simulink model "DemonstratorSimscape"  (R2020b)
settings: Solver=ode113  StartTime=0.0  StopTime=t_stop*0+20  FixedStep=1e-4
values from neighbouring files (symbols this model uses):
  brkD = 0    [main.m]
  brkI = 1e4    (= 10000)    [main.m]
  brkP = 1e5    (= 100000)    [main.m]
  d_drm = 0.5*d_drum    [main.m]
  d_shm = 0.4*d_sheave    [main.m]
  DeltaCable0 = 0    [main.m]
  Droop_scaling = 0    [main.m]
  eta_sh = 0.015    [main.m]
  filt_NUM = ones(1,200)*0.005    [main.m]
  g = 9.80665    [main.m]
  Iw = 0.5*(W.i + M.in*GB.r^2)    [main.m]
  Kp_mul = 0.3    [main.m]
  Lc0 = abs((T.ph-L.height-P.d-L.z0)*0.001)    [main.m]
  Ls1 = ((T.ph-0.5*W.pd)/1000)    [main.m]
  Ls2 = ((0.5*(T.s2+P.d)-2*P.d)/1000)    [main.m]
  M = 50e3    (= 50000)    [calcGrav.m]
  phi0_drm = -90    [main.m]
  phi0_shm = -90    [main.m]
  r_sheave = P.d*0.5    [main.m]
  s = tf('s')    [calcGrav.m]
  tau_brk = 0.001    [main.m]
  tau_em = 60e-3    (= 0.06)    [calcGrav.m]    (also in main.m)
  tau_m = tau_w/GB.r    [main.m]
  Tmax = 400e3    (= 400000)    [main.m]
  Tn_mul = 10    [main.m]
  x_drm = 0.7*r_drum    [main.m]
  x_shm = 0.7*r_sheave    [main.m]
  z0 = 0    [calcGrav.m]    (also in main.m = L.z0-P.d*0.5-P.d-P.d-L.height-T.h1-T.h2-32)
undefined symbols (not defined in the file or in its folder): C, CA, Controller_sampleTime, DiscIntNeverNeededParam, GB, L, P, Part, T, VFD_acceleration_model_factor, VFD_Adapt_factor_lower_p1458, VFD_Adapt_factor_upper_p1459, VFD_Curr_limit_var_p0641, VFD_Current_limit_p0640, VFD_Id_setp_total_r1624, VFD_Iq, VFD_Kp_n_basic_p1460, VFD_M, VFD_M_accel_T_smooth_p1517, VFD_M_lim_var_fixS_src_p1551, VFD_M_max_lower_p1521, VFD_M_max_lower_scal_p1525, VFD_M_max_up_mot_scal_p1524, VFD_M_max_upper_p1520, VFD_n_act_T_smooth_p1442, VFD_n_ctr_Kp_n_up_scal_p1461, VFD_n_ctr_Tn_n_up_sca_p1463, VFD_n_ctrl_adapt_Kp_lower_p1456, VFD_n_ctrl_adapt_Kp_upper_p1457, VFD_n_ctrl_Adpt_sig_Kp_p1455, VFD_n_ctrl_Kp_scal_p1466, VFD_n_ctrl_n_lower_p1464, VFD_n_ctrl_n_upper_p1465, VFD_n_ctrl_Tn_n_lower_p1462, VFD_n_limit_neg_p1086, VFD_n_limit_pos_p1083, VFD_n_limit_setp_p1063, VFD_n_max_p1082, VFD_n_set_filt_1_T_p1416, VFD_P_max_gen_p1531, VFD_P_max_mot_p1530, VFD_PU_I_outp_max_r0289, VFD_RFG_ramp_down_time_p1121, VFD_RFG_ramp_up_time_p1120, VFD_RFG_t_RD_scal_p1139, VFD_RFG_t_RU_scal_p1138, VSD, W, X, Y, Z
libraries: sm_lib x248, nesl_utility x128, simulink x49, pid_lib x4, cstblocks x2, simulink_extras x2
(part 5 of 10)

== system DemonstratorSimscape/Transmission System/Roof Pulley Set/Sheave_04 ==
  " " : sm_lib/Frames and Transforms/Rigid Transform  TranslationMethod=Cartesian  TranslationStandardOffset=0  TranslationLengthUnit=mm  TranslationStandardAxis=+Z  TranslationCartesianOffset=[0 -P.Bd*.25 -P.h]  TranslationROffset=0  TranslationROffsetUnits=m  TranslationZOffset=0  TranslationZOffsetUnits=m  TranslationThetaOffset=0  TranslationThetaOffsetUnits=deg  RotationMethod=ArbitraryAxis  RotationAngleUnits=deg  RotationStandardAxis=+Z  RotationAngle=90  RotationArbitraryAxis=[1 0 0]  FollAlignAxisA=+X  BaseAlignAxisA=+Y  FollAlignAxisB=+Y  BaseAlignAxisB=+Z  RotationSequenceAxes=FollowerAxes  RotationSequence=XYX  RotationSequenceAngles=[0 0 0]  RotationSequenceAnglesUnits=deg  RotationMatrix=[1 0 0; 0 1 0; 0 0 1]
  " 4" : sm_lib/Frames and Transforms/Rigid Transform  TranslationMethod=Cartesian  TranslationStandardOffset=0  TranslationLengthUnit=mm  TranslationStandardAxis=+Z  TranslationCartesianOffset=[0 -P.Bd*.25 P.h]  TranslationROffset=0  TranslationROffsetUnits=m  TranslationZOffset=0  TranslationZOffsetUnits=m  TranslationThetaOffset=0  TranslationThetaOffsetUnits=deg  RotationMethod=ArbitraryAxis  RotationAngleUnits=deg  RotationStandardAxis=+Z  RotationAngle=90  RotationArbitraryAxis=[1 0 0]  FollAlignAxisA=+X  BaseAlignAxisA=+Y  FollAlignAxisB=+Y  BaseAlignAxisB=+Z  RotationSequenceAxes=FollowerAxes  RotationSequence=XYX  RotationSequenceAngles=[0 0 0]  RotationSequenceAnglesUnits=deg  RotationMatrix=[1 0 0; 0 1 0; 0 0 1]
  PS>Sim1 : Subsystem
  Pulley 5 : sm_lib/Belts and Cables/Pulley  PitchRadius=P.Bd*0.5  PitchRadiusUnits=mm  InitialWrapAngleLowerBound=0.0  InitialWrapAngleLowerBoundUnits=deg  SenseWrapAngle=off  SensePulleyAngleA=off  SensePulleyAngleB=off  SenseFleetAngleA=off  SenseFleetAngleB=off
      settings: SourceProductBaseCode=MS
  Pulley rught red2 : Subsystem
      mask Display: image('sm_cable_drive_right_angle_pulleyA_IMAGE.png');
  Revolute Pulley5 : sm_lib/Joints/Revolute Joint  JointMode=Normal  SenseConstraintForce=on  SenseConstraintForceX=off  SenseConstraintForceY=off  SenseConstraintForceZ=off  SenseConstraintTorque=on  SenseConstraintTorqueX=off  SenseConstraintTorqueY=off  SenseConstraintTorqueZ=off  SenseTotalForce=on  SenseTotalForceX=off  SenseTotalForceY=off  SenseTotalForceZ=off  SenseTotalTorque=on  SenseTotalTorqueX=off  SenseTotalTorqueY=off  SenseTotalTorqueZ=off  CompositeWrenchDir=FollowerOnBase  CompositeWrenchFrame=BaseFrame  EquilibriumPosition=0  EquilibriumPositionUnits=deg  SpringStiffness=0  SpringStiffnessUnits=N*m/deg  DampingCoefficient=b_pulley  DampingCoefficientUnits=N*m/(deg/s)  TorqueActuationMode=NoTorque  MotionActuationMode=ComputedMotion  SensePosition=on  SenseVelocity=on  SenseAcceleration=on  SenseTorqueForce=on  SenseLowerLimitTorqueForce=off  SenseUpperLimitTorqueForce=off  LowerLimitSpecify=off  LowerLimitBound=-90  LowerLimitBoundUnits=deg  LowerLimitStiffness=1e4  LowerLimitStiffnessUnits=N*m/deg  LowerLimitDamping=10  LowerLimitDampingUnits=N*m/(deg/s)  LowerLimitTransitionRegionWidth=0.1  LowerLimitTransitionRegionWidthUnits=deg  UpperLimitSpecify=off  UpperLimitBound=90  UpperLimitBoundUnits=deg  UpperLimitStiffness=1e4  UpperLimitStiffnessUnits=N*m/deg  UpperLimitDamping=10  UpperLimitDampingUnits=N*m/(deg/s)  UpperLimitTransitionRegionWidth=0.1  UpperLimitTransitionRegionWidthUnits=deg  PositionTargetSpecify=off  PositionTargetPriority=High  PositionTargetValue=0  PositionTargetValueUnits=deg  VelocityTargetSpecify=off  VelocityTargetPriority=High  VelocityTargetValue=0  VelocityTargetValueUnits=deg/s
  ScopePulley5 : Scope  Commented=on  NumInputPorts=8
  Solid : sm_lib/Body Elements/Spherical Solid  GraphicAmbientColor=[0.15 0.15 0.15 1.0]  BasedOnType=Mass  CenterOfMass=[0 0 0]  CenterOfMassUnits=m  GraphicDiffuseColor=[0.5 0.5 0.5]  Density=1000  DensityUnits=kg/m^3  DoExposeReferenceFrame=on  GraphicEmissiveColor=[0.0 0.0 0.0 1.0]  ExportEntireGeometry=off  SerializedExposedGeometries=<ExposedGeometries/>  SerializedFrames=<Frames/>  MarkerShape=Sphere  MarkerSize=10  GraphicType=FromGeometry  InertiaType=CalculateFromGeometry  Mass=0.01  MassUnits=kg  MomentsOfInertia=[1 1 1]  MomentsOfInertiaUnits=kg*m^2  GraphicOpacity=1.0  ProductsOfInertia=[0 0 0]  ProductsOfInertiaUnits=kg*m^2  GraphicShininess=75  GraphicSpecularColor=[0.5 0.5 0.5 1.0]  SphereRadius=0.00001  SphereRadiusUnits=m  GraphicVisPropType=SimpleVisualProperties
  left face : sm_lib/Body Elements/Brick Solid  GraphicAmbientColor=[0.15 0.15 0.15 1.0]  BasedOnType=Density  BrickDimensions=[P.Bd P.h P.Bd*.5]  BrickDimensionUnits=mm  CenterOfMass=[0 0 0]  CenterOfMassUnits=m  GraphicDiffuseColor=[0.6 0.6 0.0]  Density=0  DensityUnits=g/cm^3  DoExposeReferenceFrame=on  GraphicEmissiveColor=[0.0 0.0 0.0 1.0]  ExportEntireGeometry=off  SerializedFrames=<Frames/>  MarkerShape=Sphere  MarkerSize=10  GraphicType=FromGeometry  InertiaType=CalculateFromGeometry  Mass=1  MassUnits=kg  MomentsOfInertia=[1 1 1]  MomentsOfInertiaUnits=kg*m^2  GraphicOpacity=c.opac  ProductsOfInertia=[0 0 0]  ProductsOfInertiaUnits=kg*m^2  GraphicShininess=75  GraphicSpecularColor=[0.5 0.5 0.5 1.0]  GraphicVisPropType=SimpleVisualProperties
  right face : sm_lib/Body Elements/Brick Solid  GraphicAmbientColor=[0.15 0.15 0.15 1.0]  BasedOnType=Density  BrickDimensions=[P.Bd P.h P.Bd*.5]  BrickDimensionUnits=mm  CenterOfMass=[0 0 0]  CenterOfMassUnits=m  GraphicDiffuseColor=[0.6 0.6 0.0]  Density=0  DensityUnits=g/cm^3  DoExposeReferenceFrame=on  GraphicEmissiveColor=[0.0 0.0 0.0 1.0]  ExportEntireGeometry=off  SerializedFrames=<Frames/>  MarkerShape=Sphere  MarkerSize=10  GraphicType=FromGeometry  InertiaType=CalculateFromGeometry  Mass=1  MassUnits=kg  MomentsOfInertia=[1 1 1]  MomentsOfInertiaUnits=kg*m^2  GraphicOpacity=1.0  ProductsOfInertia=[0 0 0]  ProductsOfInertiaUnits=kg*m^2  GraphicShininess=75  GraphicSpecularColor=[0.5 0.5 0.5 1.0]  GraphicVisPropType=SimpleVisualProperties
  w (rad/s) : nesl_utility/PS-Simulink Converter  PhysicalDomain=network_engine_domain  SubClassName=ps_output  LeftPortType=input  RightPortType=output  PseudoPeriodic=off  Frequencies=[]  Unit=rad/s  AffineConversion=off
  B : PMIOPort  Side=Left
  WireB : PMIOPort  Port=2  Side=Right
  WireA : PMIOPort  Port=3  Side=Right
  w5 : Outport  VectorParamsAs1DForOutWhenUnconnected=off
  wires:
  PS>Sim1/6(Out6) -> ScopePulley5/6
  PS>Sim1/3(Out3) -> ScopePulley5/3
  PS>Sim1/2(Out2) -> ScopePulley5/2
  PS>Sim1/1(Out1) -> ScopePulley5/1
  PS>Sim1/8(Out8) -> ScopePulley5/8
  PS>Sim1/7(Out7) -> ScopePulley5/7
  PS>Sim1/4(Out4) -> ScopePulley5/4
  PS>Sim1/5(Out5) -> ScopePulley5/5
  w (rad/s)/1 -> w5/1
  connections:
  " "/LConn1 -- B/RConn1 -- Revolute Pulley5/LConn1 -- " 4"/LConn1
  Solid/RConn1 -- Revolute Pulley5/RConn1 -- Pulley rught red2/LConn1
  Revolute Pulley5/RConn6 -- PS>Sim1/LConn5
  Revolute Pulley5/RConn4 -- PS>Sim1/LConn3
  Revolute Pulley5/RConn7 -- PS>Sim1/LConn6
  Revolute Pulley5/RConn5 -- PS>Sim1/LConn4
  Revolute Pulley5/RConn9 -- PS>Sim1/LConn8
  Revolute Pulley5/RConn8 -- PS>Sim1/LConn7
  Revolute Pulley5/RConn3 -- w (rad/s)/LConn1 -- PS>Sim1/LConn2
  Revolute Pulley5/RConn2 -- PS>Sim1/LConn1
  " 4"/RConn1 -- left face/RConn1
  " "/RConn1 -- right face/RConn1
  WireB/RConn1 -- Pulley 5/RConn2
  Pulley rught red2/RConn1 -- Pulley 5/LConn1
  WireA/RConn1 -- Pulley 5/RConn1

== system DemonstratorSimscape/Transmission System/Roof Pulley Set/Sheave_06 ==
  " " : sm_lib/Frames and Transforms/Rigid Transform  TranslationMethod=Cartesian  TranslationStandardOffset=0  TranslationLengthUnit=mm  TranslationStandardAxis=+Z  TranslationCartesianOffset=[0 -P.d*.25 -P.h]  TranslationROffset=0  TranslationROffsetUnits=m  TranslationZOffset=0  TranslationZOffsetUnits=m  TranslationThetaOffset=0  TranslationThetaOffsetUnits=deg  RotationMethod=ArbitraryAxis  RotationAngleUnits=deg  RotationStandardAxis=+Z  RotationAngle=90  RotationArbitraryAxis=[1 0 0]  FollAlignAxisA=+X  BaseAlignAxisA=+Y  FollAlignAxisB=+Y  BaseAlignAxisB=+Z  RotationSequenceAxes=FollowerAxes  RotationSequence=XYX  RotationSequenceAngles=[0 0 0]  RotationSequenceAnglesUnits=deg  RotationMatrix=[1 0 0; 0 1 0; 0 0 1]
  " 4" : sm_lib/Frames and Transforms/Rigid Transform  TranslationMethod=Cartesian  TranslationStandardOffset=0  TranslationLengthUnit=mm  TranslationStandardAxis=+Z  TranslationCartesianOffset=[0 -P.d*.25 P.h]  TranslationROffset=0  TranslationROffsetUnits=m  TranslationZOffset=0  TranslationZOffsetUnits=m  TranslationThetaOffset=0  TranslationThetaOffsetUnits=deg  RotationMethod=ArbitraryAxis  RotationAngleUnits=deg  RotationStandardAxis=+Z  RotationAngle=90  RotationArbitraryAxis=[1 0 0]  FollAlignAxisA=+X  BaseAlignAxisA=+Y  FollAlignAxisB=+Y  BaseAlignAxisB=+Z  RotationSequenceAxes=FollowerAxes  RotationSequence=XYX  RotationSequenceAngles=[0 0 0]  RotationSequenceAnglesUnits=deg  RotationMatrix=[1 0 0; 0 1 0; 0 0 1]
  Bending loss : Subsystem  Commented=on
  Constant : Constant  Value=g*1000
  Demux : Demux  Outputs=3
  Divide : Product  Inputs=*/
  Gain : Gain
  Gain1 : Gain  Gain=-2
  Nm : nesl_utility/Simulink-PS Converter  PhysicalDomain=network_engine_domain  SubClassName=ps_input  LeftPortType=input  RightPortType=output  PseudoPeriodic=off  Frequencies=[]  NoiseDistribution=none  NoiseParameters=[]  Unit=1  AffineConversion=off  FilteringAndDerivatives=filter  SimscapeFilterOrder=2  InputFilterTimeConstant=tau_bending  UdotUserProvided=0
  PS>Sim1 : Subsystem
  Pulley 6 : sm_lib/Belts and Cables/Pulley  PitchRadius=P.d*0.5  PitchRadiusUnits=mm  InitialWrapAngleLowerBound=0.0  InitialWrapAngleLowerBoundUnits=deg  SenseWrapAngle=off  SensePulleyAngleA=off  SensePulleyAngleB=off  SenseFleetAngleA=off  SenseFleetAngleB=off
      settings: SourceProductBaseCode=MS
  Revolute Pulley6 : sm_lib/Joints/Revolute Joint  JointMode=Normal  SenseConstraintForce=on  SenseConstraintForceX=off  SenseConstraintForceY=off  SenseConstraintForceZ=off  SenseConstraintTorque=on  SenseConstraintTorqueX=off  SenseConstraintTorqueY=off  SenseConstraintTorqueZ=off  SenseTotalForce=on  SenseTotalForceX=off  SenseTotalForceY=off  SenseTotalForceZ=off  SenseTotalTorque=on  SenseTotalTorqueX=off  SenseTotalTorqueY=off  SenseTotalTorqueZ=off  CompositeWrenchDir=FollowerOnBase  CompositeWrenchFrame=BaseFrame  EquilibriumPosition=0  EquilibriumPositionUnits=deg  SpringStiffness=0  SpringStiffnessUnits=N*m/deg  DampingCoefficient=b_pulley  DampingCoefficientUnits=N*m/(deg/s)  TorqueActuationMode=InputTorque  MotionActuationMode=ComputedMotion  SensePosition=on  SenseVelocity=on  SenseAcceleration=on  SenseTorqueForce=on  SenseLowerLimitTorqueForce=off  SenseUpperLimitTorqueForce=off  LowerLimitSpecify=off  LowerLimitBound=-90  LowerLimitBoundUnits=deg  LowerLimitStiffness=1e4  LowerLimitStiffnessUnits=N*m/deg  LowerLimitDamping=10  LowerLimitDampingUnits=N*m/(deg/s)  LowerLimitTransitionRegionWidth=0.1  LowerLimitTransitionRegionWidthUnits=deg  UpperLimitSpecify=off  UpperLimitBound=90  UpperLimitBoundUnits=deg  UpperLimitStiffness=1e4  UpperLimitStiffnessUnits=N*m/deg  UpperLimitDamping=10  UpperLimitDampingUnits=N*m/(deg/s)  UpperLimitTransitionRegionWidth=0.1  UpperLimitTransitionRegionWidthUnits=deg  PositionTargetSpecify=off  PositionTargetPriority=High  PositionTargetValue=0  PositionTargetValueUnits=deg  VelocityTargetSpecify=off  VelocityTargetPriority=High  VelocityTargetValue=0  VelocityTargetValueUnits=deg/s
  ScopePulley6 : Scope  Commented=on  NumInputPorts=8
  Sheave6 : Subsystem
      mask Display: image('sm_cable_drive_right_angle_pulleyA_IMAGE.png');
  left face : sm_lib/Body Elements/Brick Solid  GraphicAmbientColor=[0.15 0.15 0.15 1.0]  BasedOnType=Density  BrickDimensions=[P.d P.h P.d*.5]  BrickDimensionUnits=mm  CenterOfMass=[0 0 0]  CenterOfMassUnits=m  GraphicDiffuseColor=[0.6 0.6 0.0]  Density=0  DensityUnits=g/cm^3  DoExposeReferenceFrame=on  GraphicEmissiveColor=[0.0 0.0 0.0 1.0]  ExportEntireGeometry=off  SerializedFrames=<Frames/>  MarkerShape=Sphere  MarkerSize=10  GraphicType=FromGeometry  InertiaType=CalculateFromGeometry  Mass=1  MassUnits=kg  MomentsOfInertia=[1 1 1]  MomentsOfInertiaUnits=kg*m^2  GraphicOpacity=c.opac  ProductsOfInertia=[0 0 0]  ProductsOfInertiaUnits=kg*m^2  GraphicShininess=75  GraphicSpecularColor=[0.5 0.5 0.5 1.0]  GraphicVisPropType=SimpleVisualProperties
  right face : sm_lib/Body Elements/Brick Solid  GraphicAmbientColor=[0.15 0.15 0.15 1.0]  BasedOnType=Density  BrickDimensions=[P.d P.h P.d*.5]  BrickDimensionUnits=mm  CenterOfMass=[0 0 0]  CenterOfMassUnits=m  GraphicDiffuseColor=[0.6 0.6 0.0]  Density=0  DensityUnits=g/cm^3  DoExposeReferenceFrame=on  GraphicEmissiveColor=[0.0 0.0 0.0 1.0]  ExportEntireGeometry=off  SerializedFrames=<Frames/>  MarkerShape=Sphere  MarkerSize=10  GraphicType=FromGeometry  InertiaType=CalculateFromGeometry  Mass=1  MassUnits=kg  MomentsOfInertia=[1 1 1]  MomentsOfInertiaUnits=kg*m^2  GraphicOpacity=1.0  ProductsOfInertia=[0 0 0]  ProductsOfInertiaUnits=kg*m^2  GraphicShininess=75  GraphicSpecularColor=[0.5 0.5 0.5 1.0]  GraphicVisPropType=SimpleVisualProperties
  w (rad/s)1 : nesl_utility/PS-Simulink Converter  PhysicalDomain=network_engine_domain  SubClassName=ps_output  LeftPortType=input  RightPortType=output  PseudoPeriodic=off  Frequencies=[]  Unit=rad/s  AffineConversion=off
  WireA : PMIOPort  Side=Right
  Conn2 : PMIOPort  Port=2  Side=Left
  WireB : PMIOPort  Port=3  Side=Right
  w (rad/s) : Outport
  tag scope: PinLoad_R_tonne=global, S5=global, w6=global
  wires:
  [S6] -> Bending loss/1(Sin (kN))
  Bending loss/1(dT (Nm)) -> Nm/1
  Bending loss/2(Sout (kN)) -> [S5]
  Gain/1 -> Bending loss/2(w (deg/s))
  w (rad/s)1/1 -> Gain/1, [w6], w (rad/s)/1
  PS>Sim1/7(Out7) -> ScopePulley6/7
  PS>Sim1/4(Out4) -> ScopePulley6/4
  PS>Sim1/5(Out5) -> Demux/1, ScopePulley6/5
  PS>Sim1/1(Out1) -> ScopePulley6/1
  PS>Sim1/8(Out8) -> ScopePulley6/8
  PS>Sim1/2(Out2) -> ScopePulley6/2
  PS>Sim1/3(Out3) -> ScopePulley6/3
  PS>Sim1/6(Out6) -> ScopePulley6/6
  Constant/1 -> Divide/2
  Divide/1 -> [PinLoad_R_tonne]
  Demux/2 -> Gain1/1
  Gain1/1 -> Divide/1
  connections:
  WireB/RConn1 -- Pulley 6/RConn2
  Sheave6/RConn1 -- Pulley 6/LConn1
  Pulley 6/RConn1 -- WireA/RConn1
  Revolute Pulley6/LConn1 -- Conn2/RConn1 -- " "/LConn1 -- " 4"/LConn1
  PS>Sim1/LConn2 -- Revolute Pulley6/RConn3 -- w (rad/s)1/LConn1
  Revolute Pulley6/RConn4 -- PS>Sim1/LConn3
  " "/RConn1 -- right face/RConn1
  Sheave6/LConn1 -- Revolute Pulley6/RConn1
  Revolute Pulley6/RConn2 -- PS>Sim1/LConn1
  Revolute Pulley6/RConn5 -- PS>Sim1/LConn4
  Revolute Pulley6/RConn9 -- PS>Sim1/LConn8
  Revolute Pulley6/RConn8 -- PS>Sim1/LConn7
  " 4"/RConn1 -- left face/RConn1
  Revolute Pulley6/RConn6 -- PS>Sim1/LConn5
  Revolute Pulley6/RConn7 -- PS>Sim1/LConn6
  Nm/RConn1 -- Revolute Pulley6/LConn2

== system DemonstratorSimscape/Transmission System/Roof Pulley Set/Sheave_07 ==
  " " : sm_lib/Frames and Transforms/Rigid Transform  TranslationMethod=Cartesian  TranslationStandardOffset=0  TranslationLengthUnit=mm  TranslationStandardAxis=+Z  TranslationCartesianOffset=[0 -P.d*.25 -P.h]  TranslationROffset=0  TranslationROffsetUnits=m  TranslationZOffset=0  TranslationZOffsetUnits=m  TranslationThetaOffset=0  TranslationThetaOffsetUnits=deg  RotationMethod=ArbitraryAxis  RotationAngleUnits=deg  RotationStandardAxis=+Z  RotationAngle=90  RotationArbitraryAxis=[1 0 0]  FollAlignAxisA=+X  BaseAlignAxisA=+Y  FollAlignAxisB=+Y  BaseAlignAxisB=+Z  RotationSequenceAxes=FollowerAxes  RotationSequence=XYX  RotationSequenceAngles=[0 0 0]  RotationSequenceAnglesUnits=deg  RotationMatrix=[1 0 0; 0 1 0; 0 0 1]
  " 4" : sm_lib/Frames and Transforms/Rigid Transform  TranslationMethod=Cartesian  TranslationStandardOffset=0  TranslationLengthUnit=mm  TranslationStandardAxis=+Z  TranslationCartesianOffset=[0 -P.d*.25 P.h]  TranslationROffset=0  TranslationROffsetUnits=m  TranslationZOffset=0  TranslationZOffsetUnits=m  TranslationThetaOffset=0  TranslationThetaOffsetUnits=deg  RotationMethod=ArbitraryAxis  RotationAngleUnits=deg  RotationStandardAxis=+Z  RotationAngle=90  RotationArbitraryAxis=[1 0 0]  FollAlignAxisA=+X  BaseAlignAxisA=+Y  FollAlignAxisB=+Y  BaseAlignAxisB=+Z  RotationSequenceAxes=FollowerAxes  RotationSequence=XYX  RotationSequenceAngles=[0 0 0]  RotationSequenceAnglesUnits=deg  RotationMatrix=[1 0 0; 0 1 0; 0 0 1]
  Bending loss : Subsystem  Commented=on
  Gain : Gain
  Nm : nesl_utility/Simulink-PS Converter  PhysicalDomain=network_engine_domain  SubClassName=ps_input  LeftPortType=input  RightPortType=output  PseudoPeriodic=off  Frequencies=[]  NoiseDistribution=none  NoiseParameters=[]  Unit=1  AffineConversion=off  FilteringAndDerivatives=filter  SimscapeFilterOrder=2  InputFilterTimeConstant=tau_bending  UdotUserProvided=0
  PS>Sim1 : Subsystem
  Pulley 7 : sm_lib/Belts and Cables/Pulley  PitchRadius=P.d*0.5  PitchRadiusUnits=mm  InitialWrapAngleLowerBound=0.0  InitialWrapAngleLowerBoundUnits=deg  SenseWrapAngle=off  SensePulleyAngleA=off  SensePulleyAngleB=off  SenseFleetAngleA=off  SenseFleetAngleB=off
      settings: SourceProductBaseCode=MS
  Revolute Pulley7 : sm_lib/Joints/Revolute Joint  JointMode=Normal  SenseConstraintForce=on  SenseConstraintForceX=off  SenseConstraintForceY=off  SenseConstraintForceZ=off  SenseConstraintTorque=on  SenseConstraintTorqueX=off  SenseConstraintTorqueY=off  SenseConstraintTorqueZ=off  SenseTotalForce=on  SenseTotalForceX=off  SenseTotalForceY=off  SenseTotalForceZ=off  SenseTotalTorque=on  SenseTotalTorqueX=off  SenseTotalTorqueY=off  SenseTotalTorqueZ=off  CompositeWrenchDir=FollowerOnBase  CompositeWrenchFrame=BaseFrame  EquilibriumPosition=0  EquilibriumPositionUnits=deg  SpringStiffness=0  SpringStiffnessUnits=N*m/deg  DampingCoefficient=b_pulley  DampingCoefficientUnits=N*m/(deg/s)  TorqueActuationMode=InputTorque  MotionActuationMode=ComputedMotion  SensePosition=on  SenseVelocity=on  SenseAcceleration=on  SenseTorqueForce=on  SenseLowerLimitTorqueForce=off  SenseUpperLimitTorqueForce=off  LowerLimitSpecify=off  LowerLimitBound=-90  LowerLimitBoundUnits=deg  LowerLimitStiffness=1e4  LowerLimitStiffnessUnits=N*m/deg  LowerLimitDamping=10  LowerLimitDampingUnits=N*m/(deg/s)  LowerLimitTransitionRegionWidth=0.1  LowerLimitTransitionRegionWidthUnits=deg  UpperLimitSpecify=off  UpperLimitBound=90  UpperLimitBoundUnits=deg  UpperLimitStiffness=1e4  UpperLimitStiffnessUnits=N*m/deg  UpperLimitDamping=10  UpperLimitDampingUnits=N*m/(deg/s)  UpperLimitTransitionRegionWidth=0.1  UpperLimitTransitionRegionWidthUnits=deg  PositionTargetSpecify=off  PositionTargetPriority=High  PositionTargetValue=0  PositionTargetValueUnits=deg  VelocityTargetSpecify=off  VelocityTargetPriority=High  VelocityTargetValue=0  VelocityTargetValueUnits=deg/s
  ScopePulley7 : Scope  Commented=on  NumInputPorts=8
  Sheave7 : Subsystem
      mask Display: image('sm_cable_drive_right_angle_pulleyA_IMAGE.png');
  left face : sm_lib/Body Elements/Brick Solid  GraphicAmbientColor=[0.15 0.15 0.15 1.0]  BasedOnType=Density  BrickDimensions=[P.d P.h P.d*.5]  BrickDimensionUnits=mm  CenterOfMass=[0 0 0]  CenterOfMassUnits=m  GraphicDiffuseColor=[0.6 0.6 0.0]  Density=0  DensityUnits=g/cm^3  DoExposeReferenceFrame=on  GraphicEmissiveColor=[0.0 0.0 0.0 1.0]  ExportEntireGeometry=off  SerializedFrames=<Frames/>  MarkerShape=Sphere  MarkerSize=10  GraphicType=FromGeometry  InertiaType=CalculateFromGeometry  Mass=1  MassUnits=kg  MomentsOfInertia=[1 1 1]  MomentsOfInertiaUnits=kg*m^2  GraphicOpacity=c.opac  ProductsOfInertia=[0 0 0]  ProductsOfInertiaUnits=kg*m^2  GraphicShininess=75  GraphicSpecularColor=[0.5 0.5 0.5 1.0]  GraphicVisPropType=SimpleVisualProperties
  right face : sm_lib/Body Elements/Brick Solid  GraphicAmbientColor=[0.15 0.15 0.15 1.0]  BasedOnType=Density  BrickDimensions=[P.d P.h P.d*.5]  BrickDimensionUnits=mm  CenterOfMass=[0 0 0]  CenterOfMassUnits=m  GraphicDiffuseColor=[0.6 0.6 0.0]  Density=0  DensityUnits=g/cm^3  DoExposeReferenceFrame=on  GraphicEmissiveColor=[0.0 0.0 0.0 1.0]  ExportEntireGeometry=off  SerializedFrames=<Frames/>  MarkerShape=Sphere  MarkerSize=10  GraphicType=FromGeometry  InertiaType=CalculateFromGeometry  Mass=1  MassUnits=kg  MomentsOfInertia=[1 1 1]  MomentsOfInertiaUnits=kg*m^2  GraphicOpacity=1.0  ProductsOfInertia=[0 0 0]  ProductsOfInertiaUnits=kg*m^2  GraphicShininess=75  GraphicSpecularColor=[0.5 0.5 0.5 1.0]  GraphicVisPropType=SimpleVisualProperties
  w (rad/s)0 : nesl_utility/PS-Simulink Converter  PhysicalDomain=network_engine_domain  SubClassName=ps_output  LeftPortType=input  RightPortType=output  PseudoPeriodic=off  Frequencies=[]  Unit=rad/s  AffineConversion=off
  Conn1 : PMIOPort  Side=Left
  Conn2 : PMIOPort  Port=2  Side=Right
  Conn3 : PMIOPort  Port=3  Side=Right
  w (rad/s) : Outport
  tag scope: S6=global, w7=global
  wires:
  [S7] -> Bending loss/1(Sin (kN))
  Bending loss/1(dT (Nm)) -> Nm/1
  Bending loss/2(Sout (kN)) -> [S6]
  Gain/1 -> Bending loss/2(w (deg/s))
  PS>Sim1/8(Out8) -> ScopePulley7/8
  PS>Sim1/1(Out1) -> ScopePulley7/1
  PS>Sim1/2(Out2) -> ScopePulley7/2
  PS>Sim1/3(Out3) -> ScopePulley7/3
  PS>Sim1/5(Out5) -> ScopePulley7/5
  w (rad/s)0/1 -> [w7], Gain/1, w (rad/s)/1
  PS>Sim1/4(Out4) -> ScopePulley7/4
  PS>Sim1/7(Out7) -> ScopePulley7/7
  PS>Sim1/6(Out6) -> ScopePulley7/6
  connections:
  Sheave7/RConn1 -- Pulley 7/LConn1
  Pulley 7/RConn1 -- Conn2/RConn1
  Conn3/RConn1 -- Pulley 7/RConn2
  PS>Sim1/LConn2 -- Revolute Pulley7/RConn3 -- w (rad/s)0/LConn1
  Revolute Pulley7/LConn1 -- Conn1/RConn1 -- " "/LConn1 -- " 4"/LConn1
  Sheave7/LConn1 -- Revolute Pulley7/RConn1
  Revolute Pulley7/RConn2 -- PS>Sim1/LConn1
  Revolute Pulley7/RConn6 -- PS>Sim1/LConn5
  Revolute Pulley7/RConn8 -- PS>Sim1/LConn7
  Revolute Pulley7/RConn5 -- PS>Sim1/LConn4
  Revolute Pulley7/RConn7 -- PS>Sim1/LConn6
  Revolute Pulley7/RConn9 -- PS>Sim1/LConn8
  " "/RConn1 -- right face/RConn1
  " 4"/RConn1 -- left face/RConn1
  Revolute Pulley7/RConn4 -- PS>Sim1/LConn3
  Nm/RConn1 -- Revolute Pulley7/LConn2

== system DemonstratorSimscape/Visualization/System Powers/Power and Efficiency ==
  MotSpdL (rpm) : Inport
  MotTrqL (Nm) : Inport  Port=2
  MotSpdR (rpm) : Inport  Port=3
  MotTrqR (Nm) : Inport  Port=4
  Gain7 : Gain  Gain=pi/30
  Gain8 : Gain  Gain=pi/30
  Lumped Efficiency Left : Subsystem
  Lumped Efficiency Right : Subsystem
  Product2 : Product
  Product3 : Product
  Sum : Sum
  Sum2 : Sum
  kW : Gain  Gain=1e-3
  kW1 : Gain  Gain=1e-3
  MechPwr_kW : Outport
  ElecPwr_kW : Outport  Port=2
  wires:
  MotTrqL (Nm)/1 -> Product3/2
  Product3/1 -> Sum/1, Lumped Efficiency Left/2(mech power [W])
  MotSpdR (rpm)/1 -> Lumped Efficiency Right/1(motor speed [rpm]), Gain7/1
  Sum/1 -> kW/1
  Gain7/1 -> Product2/1
  Product2/1 -> Lumped Efficiency Right/2(mech power [W]), Sum/2
  MotTrqR (Nm)/1 -> Product2/2
  MotSpdL (rpm)/1 -> Lumped Efficiency Left/1(motor speed [rpm]), Gain8/1
  Gain8/1 -> Product3/1
  Lumped Efficiency Left/1(elec power (W)) -> Sum2/1
  Lumped Efficiency Right/1(elec power (W)) -> Sum2/2
  Sum2/1 -> kW1/1
  kW/1 -> MechPwr_kW/1
  kW1/1 -> ElecPwr_kW/1

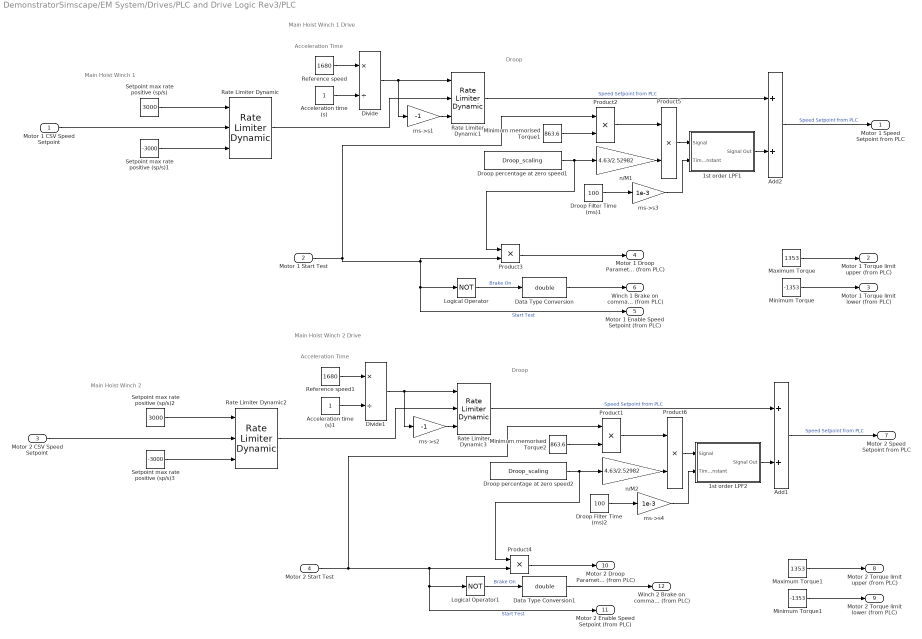
== system DemonstratorSimscape/EM System/Drives/PLC and Drive Logic Rev3/PLC ==
  note: Main Hoist Winch 1 Drive
  note: Acceleration Time
  note: Droop
  note: Main Hoist Winch 1
  note: Main Hoist Winch 2 Drive
  note: Acceleration Time
  note: Droop
  note: Main Hoist Winch 2
  Motor 1 CSV Speed Setpoint : Inport
  Motor 1 Start Test : Inport  Port=2
  Motor 2 CSV Speed Setpoint : Inport  Port=3
  Motor 2 Start Test : Inport  Port=4
  1st order LPF1 : Subsystem  mask{time_constant=0.1, Yo=0}
      mask prompts: time_constant "Time Constant (s)"; Yo "Initial Condition"
  1st order LPF2 : Subsystem  mask{time_constant=0.1, Yo=0}
      mask prompts: time_constant "Time Constant (s)"; Yo "Initial Condition"
  Acceleration time (s) : Constant
  Acceleration time (s)1 : Constant
  Add1 : Sum
  Add2 : Sum
  Data Type Conversion : DataTypeConversion  OutDataTypeStr=double
  Data Type Conversion1 : DataTypeConversion  OutDataTypeStr=double
  Divide : Product  Inputs=*/
  Divide1 : Product  Inputs=*/
  Droop Filter Time (ms)1 : Constant  Value=100
  Droop Filter Time (ms)2 : Constant  Value=100
  Droop percentage at zero speed1 : Constant  Value=Droop_scaling
  Droop percentage at zero speed2 : Constant  Value=Droop_scaling
  Logical Operator : Logic  Operator=NOT  AllPortsSameDT=off  OutDataTypeStr=boolean
  Logical Operator1 : Logic  Operator=NOT  AllPortsSameDT=off  OutDataTypeStr=boolean
  Maximum Torque : Constant  Value=1353
  Maximum Torque1 : Constant  Value=1353
  Minimum Torque : Constant  Value=-1353
  Minimum Torque1 : Constant  Value=-1353
  Minimum memorised Torque1 : Constant  Value=863.6
  Minimum memorised Torque2 : Constant  Value=863.6
  Product{1..2,5..6} (4 alike) : Product  Inputs=**
  Product3 : Product
  Product4 : Product
  Rate Limiter Dynamic{,1..3} (4 alike) : simulink/Discontinuities/Rate Limiter Dynamic
  Reference speed : Constant  Value=1680
  Reference speed1 : Constant  Value=1680
  Setpoint max rate positive (sp/s) : Constant  Value=3000
  Setpoint max rate positive (sp/s)1 : Constant  Value=-3000
  Setpoint max rate positive (sp/s)2 : Constant  Value=3000
  Setpoint max rate positive (sp/s)3 : Constant  Value=-3000
  ms->s1 : Gain  Gain=-1
  ms->s2 : Gain  Gain=-1
  ms->s3 : Gain  Gain=1e-3
  ms->s4 : Gain  Gain=1e-3
  n/M1 : Gain  Gain=4.63/2.52982
  n/M2 : Gain  Gain=4.63/2.52982
  Motor 1 Speed Setpoint from PLC : Outport
  Motor 1 Torque limit upper (from PLC) : Outport  Port=2
  Motor 1 Torque limit lower (from PLC) : Outport  Port=3
  Motor 1 Droop Parameter (from PLC) : Outport  Port=4
  Motor 1 Enable Speed Setpoint (from PLC) : Outport  Port=5
  Winch 1 Brake on command (from PLC) : Outport  Port=6
  Motor 2 Speed Setpoint from PLC : Outport  Port=7
  Motor 2 Torque limit upper (from PLC) : Outport  Port=8
  Motor 2 Torque limit lower (from PLC) : Outport  Port=9
  Motor 2 Droop Parameter (from PLC) : Outport  Port=10
  Motor 2 Enable Speed Setpoint (from PLC) : Outport  Port=11
  Winch 2 Brake on command (from PLC) : Outport  Port=12
  wires:
  Product2/1 -> Product5/1
  n/M1/1 -> Product5/2
  ms->s1/1 -> Rate Limiter Dynamic1/3
  ms->s3/1 -> 1st order LPF1/2(Time Constant)
  Divide/1 -> ms->s1/1, Rate Limiter Dynamic1/1
  Setpoint max rate positive (sp/s)/1 -> Rate Limiter Dynamic/1
  Setpoint max rate positive (sp/s)1/1 -> Rate Limiter Dynamic/3
  Product5/1 -> 1st order LPF1/1(Signal)
  Droop Filter Time (ms)1/1 -> ms->s3/1
  1st order LPF1/1(Signal Out) -> Add2/2
  Droop percentage at zero speed1/1 -> Product3/1, n/M1/1
  Rate Limiter Dynamic/1 -> Rate Limiter Dynamic1/2
  Minimum memorised Torque1/1 -> Product2/2
  Reference speed/1 -> Divide/1
  Acceleration time (s)/1 -> Divide/2
  Add2/1 -> Motor 1 Speed Setpoint from PLC/1  "Speed Setpoint from PLC"
  Maximum Torque/1 -> Motor 1 Torque limit upper (from PLC)/1
  Minimum Torque/1 -> Motor 1 Torque limit lower (from PLC)/1
  Rate Limiter Dynamic1/1 -> Add2/1  "Speed Setpoint from PLC"
  Motor 1 Start Test/1 -> Motor 1 Enable Speed Setpoint (from PLC)/1, Logical Operator/1, Product3/2, Product2/1  "Start Test"
  Product3/1 -> Motor 1 Droop Parameter (from PLC)/1
  Logical Operator/1 -> Data Type Conversion/1  "Brake On"
  Data Type Conversion/1 -> Winch 1 Brake on command (from PLC)/1
  Motor 1 CSV Speed Setpoint/1 -> Rate Limiter Dynamic/2
  Motor 2 CSV Speed Setpoint/1 -> Rate Limiter Dynamic2/2
  Data Type Conversion1/1 -> Winch 2 Brake on command (from PLC)/1
  Logical Operator1/1 -> Data Type Conversion1/1  "Brake On"
  Product4/1 -> Motor 2 Droop Parameter (from PLC)/1
  Motor 2 Start Test/1 -> Product1/1, Motor 2 Enable Speed Setpoint (from PLC)/1, Logical Operator1/1, Product4/2  "Start Test"
  Rate Limiter Dynamic3/1 -> Add1/1  "Speed Setpoint from PLC"
  Minimum Torque1/1 -> Motor 2 Torque limit lower (from PLC)/1
  Maximum Torque1/1 -> Motor 2 Torque limit upper (from PLC)/1
  Add1/1 -> Motor 2 Speed Setpoint from PLC/1  "Speed Setpoint from PLC"
  Acceleration time (s)1/1 -> Divide1/2
  Reference speed1/1 -> Divide1/1
  Minimum memorised Torque2/1 -> Product1/2
  Rate Limiter Dynamic2/1 -> Rate Limiter Dynamic3/2
  Droop percentage at zero speed2/1 -> n/M2/1, Product4/1
  1st order LPF2/1(Signal Out) -> Add1/2
  Droop Filter Time (ms)2/1 -> ms->s4/1
  Product6/1 -> 1st order LPF2/1(Signal)
  Setpoint max rate positive (sp/s)3/1 -> Rate Limiter Dynamic2/3
  Setpoint max rate positive (sp/s)2/1 -> Rate Limiter Dynamic2/1
  Divide1/1 -> Rate Limiter Dynamic3/1, ms->s2/1
  ms->s4/1 -> 1st order LPF2/2(Time Constant)
  ms->s2/1 -> Rate Limiter Dynamic3/3
  n/M2/1 -> Product6/2
  Product1/1 -> Product6/1

== system DemonstratorSimscape/EM System/Drives/PLC and Drive Logic Rev3/VFD Control1 ==
  Measured RPM : Inport
  "[p1070(0)] Main Setpoint (Speed setpoint from PLC)" : Inport  Port=2
  "[p1522] Torque limit upper (from PLC)" : Inport  Port=3
  "[p1523] Torque limit lower (from PLC)" : Inport  Port=4
  "[p21501] Droop Parameter from PLC" : Inport  Port=5
  Enable Speed Controller : Inport  Port=6
  WAB Mode : Inport  Port=7
  WAB Mode Speed_Controller Setpoint (r1438) : Inport  Port=8
  Bus Creator : BusCreator  Inputs=12
  "[3001] Setpoint Channel " : Subsystem
  "[6020] Speed control and generation of the torque limits " : Subsystem
  "[r0079] M_set total (Torque setpoint)" : Outport  VectorParamsAs1DForOutWhenUnconnected=off
  Motor 1 Diagnostics Bus : Outport  Port=2
  wires:
  "[6020] Speed control and generation of the torque limits "/12("[r1539] Lower effective torque limit") -> Bus Creator/11  "[r1539] Lower effective torque limit"
  "[6020] Speed control and generation of the torque limits "/11("[r1538] Upper effective torque limit") -> Bus Creator/10  "[r1538] Upper effective torque limit"
  "[6020] Speed control and generation of the torque limits "/10("[r1508] Torque setpoint before supplementary torque") -> Bus Creator/9  "[r1508] Torque setpoint before supplementary torque"
  "[6020] Speed control and generation of the torque limits "/9("[r1516] Supplementary torque and acceleration torque ") -> Bus Creator/8  "[r1516] Supplementary torque and acceleration torque"
  "[6020] Speed control and generation of the torque limits "/8("[r1480] Speed Controller PI torque Output") -> Bus Creator/7  "[r1480] Speed Controller PI torque Output"
  "[6020] Speed control and generation of the torque limits "/7("[r64] Speed controller system deviation") -> Bus Creator/6  "[r64] Speed controller system deviation"
  "[6020] Speed control and generation of the torque limits "/6("[r1469] Speed Controller integral time effective") -> Bus Creator/5  "[r1469] Speed Controller integral time effective"
  "[6020] Speed control and generation of the torque limits "/5("[r1468] Speed Controller P-gain effective") -> Bus Creator/4  "[r1468] Speed Controller P-gain effective"
  Bus Creator/1 -> Motor 1 Diagnostics Bus/1
  WAB Mode Speed_Controller Setpoint (r1438)/1 -> "[6020] Speed control and generation of the torque limits "/10("[r1438] Speed controller speed setpoint")
  WAB Mode/1 -> "[6020] Speed control and generation of the torque limits "/9(WAB Mode)
  "[6020] Speed control and generation of the torque limits "/2("[r1482] Speed Controller I torque Output") -> Bus Creator/1  "[r1482] Speed Controller I torque Output"
  "[6020] Speed control and generation of the torque limits "/3("[r1481] Speed Controller P torque Output") -> Bus Creator/2  "[r1481] Speed Controller P torque Output"
  Measured RPM/1 -> "[6020] Speed control and generation of the torque limits "/1("[r63[0]] Speed actual value, unsmoothed")
  "[p1070(0)] Main Setpoint (Speed setpoint from PLC)"/1 -> Bus Creator/12, "[3001] Setpoint Channel "/1("[p1070(0)] Main Setpoint")  "[p1070(0)] Main Setpoint (Speed setpoint from PLC)"
  "[3001] Setpoint Channel "/1("[r1170] n_ctrl setp sum (Speed setpoint after the RFG)") -> "[6020] Speed control and generation of the torque limits "/2("[r1170] n_ctrl setp sum (Speed setpoint after the RFG)")
  "[3001] Setpoint Channel "/2("[r1084] n_limit pos eff Positive Speed limit (rpm)") -> "[6020] Speed control and generation of the torque limits "/3("[r1084] n_limit pos eff Positive Speed limit (rpm)")
  "[3001] Setpoint Channel "/3("[r1087] n_limit neg eff Negative Speed limit (rpm)") -> "[6020] Speed control and generation of the torque limits "/4("[r1087] n_limit neg eff Negative Speed limit (rpm)")
  "[6020] Speed control and generation of the torque limits "/4(Speed setpoint (into speed controller)) -> Bus Creator/3  "Speed setpoint (into speed controller)"
  "[6020] Speed control and generation of the torque limits "/1("[r0079] M_set total (Torque setpoint)") -> "[r0079] M_set total (Torque setpoint)"/1
  "[p1523] Torque limit lower (from PLC)"/1 -> "[6020] Speed control and generation of the torque limits "/6("[p1523] Torque limit lower (from PLC)")
  "[p1522] Torque limit upper (from PLC)"/1 -> "[6020] Speed control and generation of the torque limits "/5("[p1522] Torque limit upper (from PLC)")
  "[p21501] Droop Parameter from PLC"/1 -> "[6020] Speed control and generation of the torque limits "/7("[p21501] Droop Parameter from PLC")
  Enable Speed Controller/1 -> "[6020] Speed control and generation of the torque limits "/8(Enable Speed Controller)

== system DemonstratorSimscape/EM System/Drives/PLC and Drive Logic Rev3/VFD Control2 ==
  Measured RPM : Inport
  "[p1070(0)] Main Setpoint (Speed setpoint from PLC)" : Inport  Port=2
  "[p1522] Torque limit upper (from PLC)" : Inport  Port=3
  "[p1523] Torque limit lower (from PLC)" : Inport  Port=4
  "[p21501] Droop Parameter from PLC" : Inport  Port=5
  Enable Speed Controller : Inport  Port=6
  WAB Mode : Inport  Port=7
  WAB Mode Speed_Controller Setpoint (r1438) : Inport  Port=8
  Bus Creator : BusCreator  Inputs=12
  "[3001] Setpoint Channel " : Subsystem
  "[6020] Speed control and generation of the torque limits " : Subsystem
  "[r0079] M_set total (Torque setpoint)" : Outport  VectorParamsAs1DForOutWhenUnconnected=off
  Motor 1 Diagnostics Bus : Outport  Port=2
  wires:
  "[6020] Speed control and generation of the torque limits "/12("[r1539] Lower effective torque limit") -> Bus Creator/11  "[r1539] Lower effective torque limit"
  "[6020] Speed control and generation of the torque limits "/11("[r1538] Upper effective torque limit") -> Bus Creator/10  "[r1538] Upper effective torque limit"
  "[6020] Speed control and generation of the torque limits "/10("[r1508] Torque setpoint before supplementary torque") -> Bus Creator/9  "[r1508] Torque setpoint before supplementary torque"
  "[6020] Speed control and generation of the torque limits "/9("[r1516] Supplementary torque and acceleration torque ") -> Bus Creator/8  "[r1516] Supplementary torque and acceleration torque"
  "[6020] Speed control and generation of the torque limits "/8("[r1480] Speed Controller PI torque Output") -> Bus Creator/7  "[r1480] Speed Controller PI torque Output"
  "[6020] Speed control and generation of the torque limits "/7("[r64] Speed controller system deviation") -> Bus Creator/6  "[r64] Speed controller system deviation"
  "[6020] Speed control and generation of the torque limits "/6("[r1469] Speed Controller integral time effective") -> Bus Creator/5  "[r1469] Speed Controller integral time effective"
  "[6020] Speed control and generation of the torque limits "/5("[r1468] Speed Controller P-gain effective") -> Bus Creator/4  "[r1468] Speed Controller P-gain effective"
  Bus Creator/1 -> Motor 1 Diagnostics Bus/1
  WAB Mode Speed_Controller Setpoint (r1438)/1 -> "[6020] Speed control and generation of the torque limits "/10("[r1438] Speed controller speed setpoint")
  WAB Mode/1 -> "[6020] Speed control and generation of the torque limits "/9(WAB Mode)
  "[6020] Speed control and generation of the torque limits "/2("[r1482] Speed Controller I torque Output") -> Bus Creator/1  "[r1482] Speed Controller I torque Output"
  "[6020] Speed control and generation of the torque limits "/3("[r1481] Speed Controller P torque Output") -> Bus Creator/2  "[r1481] Speed Controller P torque Output"
  Measured RPM/1 -> "[6020] Speed control and generation of the torque limits "/1("[r63[0]] Speed actual value, unsmoothed")
  "[p1070(0)] Main Setpoint (Speed setpoint from PLC)"/1 -> Bus Creator/12, "[3001] Setpoint Channel "/1("[p1070(0)] Main Setpoint")  "[p1070(0)] Main Setpoint (Speed setpoint from PLC)"
  "[3001] Setpoint Channel "/1("[r1170] n_ctrl setp sum (Speed setpoint after the RFG)") -> "[6020] Speed control and generation of the torque limits "/2("[r1170] n_ctrl setp sum (Speed setpoint after the RFG)")
  "[3001] Setpoint Channel "/2("[r1084] n_limit pos eff Positive Speed limit (rpm)") -> "[6020] Speed control and generation of the torque limits "/3("[r1084] n_limit pos eff Positive Speed limit (rpm)")
  "[3001] Setpoint Channel "/3("[r1087] n_limit neg eff Negative Speed limit (rpm)") -> "[6020] Speed control and generation of the torque limits "/4("[r1087] n_limit neg eff Negative Speed limit (rpm)")
  "[6020] Speed control and generation of the torque limits "/4(Speed setpoint (into speed controller)) -> Bus Creator/3  "Speed setpoint (into speed controller)"
  "[6020] Speed control and generation of the torque limits "/1("[r0079] M_set total (Torque setpoint)") -> "[r0079] M_set total (Torque setpoint)"/1
  "[p1523] Torque limit lower (from PLC)"/1 -> "[6020] Speed control and generation of the torque limits "/6("[p1523] Torque limit lower (from PLC)")
  "[p1522] Torque limit upper (from PLC)"/1 -> "[6020] Speed control and generation of the torque limits "/5("[p1522] Torque limit upper (from PLC)")
  "[p21501] Droop Parameter from PLC"/1 -> "[6020] Speed control and generation of the torque limits "/7("[p21501] Droop Parameter from PLC")
  Enable Speed Controller/1 -> "[6020] Speed control and generation of the torque limits "/8(Enable Speed Controller)

== system DemonstratorSimscape/EM System/Drives/Simple Drive Model/Pwr Limits (R) ==
  Spd : Inport  SampleTime=C.ts
  TrqIn : Inport  Port=2
  Limits : Subsystem
  No Limits : Subsystem  Commented=on
  TrqSat : Outport
  wires:
  Spd/1 -> Limits/2(MotSpd (rpm))
  TrqIn/1 -> Limits/1(TrqIn (Nm)), No Limits/1(TrqIn (Nm))
  Limits/1(TrqSat (Nm)) -> TrqSat/1

== system DemonstratorSimscape/EM System/Drives/Simple Drive Model/Spd Limits1 ==
  SpdIn : Inport
  DerSatInt : Subsystem  Commented=on
  Mux1 : Mux  Commented=on  Inputs=3
  Mux2 : Mux  Commented=on  Inputs=3
  No Rate Limits : Subsystem
  Rate Limiter : Subsystem  Commented=on
  der : Scope  Commented=on  NumInputPorts=2
  SpdLim : Outport
  wires:
  Rate Limiter/2(RateSat) -> Mux2/3
  DerSatInt/2(RateSat) -> Mux2/2
  Rate Limiter/1(SpdLim) -> Mux1/3
  DerSatInt/1(SpdLim) -> Mux1/2
  DerSatInt/3(Rate) -> Mux2/1
  No Rate Limits/1(SpdLim) -> SpdLim/1
  SpdIn/1 -> No Rate Limits/1(SpdIn), DerSatInt/1(SpdIn), Rate Limiter/1(SpdIn), Mux1/1
  Mux2/1 -> der/2
  Mux1/1 -> der/1

== system DemonstratorSimscape/EM System/Drives/Simple Drive Model1/Pwr Limits (L) ==
  Spd : Inport  SampleTime=C.ts
  TrqIn : Inport  Port=2
  Limits : Subsystem
  No Limits : Subsystem  Commented=on
  TrqSat : Outport
  wires:
  Limits/1(TrqSat (Nm)) -> TrqSat/1
  Spd/1 -> Limits/2(MotSpd (rpm))
  TrqIn/1 -> Limits/1(TrqIn (Nm)), No Limits/1(TrqIn (Nm))

== system DemonstratorSimscape/EM System/Drives/Simple Drive Model1/Pwr Limits (R) ==
  Spd : Inport  SampleTime=C.ts
  TrqIn : Inport  Port=2
  Limits : Subsystem
  No Limits : Subsystem  Commented=on
  TrqSat : Outport
  wires:
  Limits/1(TrqSat (Nm)) -> TrqSat/1
  TrqIn/1 -> No Limits/1(TrqIn (Nm)), Limits/1(TrqIn (Nm))
  Spd/1 -> Limits/2(MotSpd (rpm))

== system DemonstratorSimscape/EM System/Drives/Simple Drive Model1/Spd Limits ==
  SpdIn : Inport
  DerSatInt : Subsystem  Commented=on
  Mux1 : Mux  Commented=on  Inputs=3
  Mux2 : Mux  Commented=on  Inputs=3
  No Rate Limits : Subsystem
  Rate Limiter : Subsystem  Commented=on
  der : Scope  Commented=on  NumInputPorts=2
  SpdLim : Outport
  wires:
  Rate Limiter/2(RateSat) -> Mux2/3
  DerSatInt/2(RateSat) -> Mux2/2
  Rate Limiter/1(SpdLim) -> Mux1/3
  DerSatInt/1(SpdLim) -> Mux1/2
  DerSatInt/3(Rate) -> Mux2/1
  No Rate Limits/1(SpdLim) -> SpdLim/1
  SpdIn/1 -> No Rate Limits/1(SpdIn), DerSatInt/1(SpdIn), Rate Limiter/1(SpdIn), Mux1/1
  Mux2/1 -> der/2
  Mux1/1 -> der/1

== system DemonstratorSimscape/EM System/Drives/Simple Drive Model1/Spd Limits1 ==
  SpdIn : Inport
  DerSatInt : Subsystem  Commented=on
  Mux1 : Mux  Commented=on  Inputs=3
  Mux2 : Mux  Commented=on  Inputs=3
  No Rate Limits : Subsystem
  Rate Limiter : Subsystem  Commented=on
  der : Scope  Commented=on  NumInputPorts=2
  SpdLim : Outport
  wires:
  Mux1/1 -> der/1
  Mux2/1 -> der/2
  SpdIn/1 -> Mux1/1, Rate Limiter/1(SpdIn), DerSatInt/1(SpdIn), No Rate Limits/1(SpdIn)
  No Rate Limits/1(SpdLim) -> SpdLim/1
  DerSatInt/3(Rate) -> Mux2/1
  DerSatInt/1(SpdLim) -> Mux1/2
  Rate Limiter/1(SpdLim) -> Mux1/3
  DerSatInt/2(RateSat) -> Mux2/2
  Rate Limiter/2(RateSat) -> Mux2/3

== system DemonstratorSimscape/EM System/Motor Winch Left/Gearbox/Gearbox efficiency ==
  MotTrqRef : Inport
  MotSpd : Inport  Port=2
  Divide : Product  Inputs=**
  Gain : Gain  Gain=-1
  Power : Math  Operator=pow  SaturateOnIntegerOverflow=on
  Sign1 : Signum
  gearbox efficiency : Constant  Value=GB.eff
  WinchTrq : Outport
  wires:
  Power/1 -> Divide/2
  Divide/1 -> WinchTrq/1
  MotTrqRef/1 -> Divide/1
  gearbox efficiency/1 -> Power/1
  Gain/1 -> Sign1/1
  Sign1/1 -> Power/2
  MotSpd/1 -> Gain/1

== system DemonstratorSimscape/EM System/Motor Winch Left/Gearbox/Sheaves efficiency ==
  WinchTrq : Inport
  MotSpd : Inport  Port=2
  Divide : Product  Inputs=**
  Gain : Gain  Gain=-1
  Power : Math  Operator=pow  SaturateOnIntegerOverflow=on
  Sign : Signum
  combined sheaves efficiency : Constant  Value=P.eff
  swSheavesEff : ManualSwitch  CurrentSetting=0
  WinchTrq' : Outport
  wires:
  Power/1 -> Divide/2
  Sign/1 -> Power/2
  WinchTrq/1 -> Divide/1, swSheavesEff/1
  Gain/1 -> Sign/1
  MotSpd/1 -> Gain/1
  combined sheaves efficiency/1 -> Power/1
  Divide/1 -> swSheavesEff/2
  swSheavesEff/1 -> WinchTrq'/1

== system DemonstratorSimscape/EM System/Motor Winch Left/Motor/Ideal motor ==
  MotTrqRef : Inport
  MotSpd : Inport  Port=2
  MotTrq : Outport
  wires:
  MotTrqRef/1 -> MotTrq/1

== system DemonstratorSimscape/EM System/Motor Winch Left/Motor/Motor dynamics ==
  TrqIn : Inport
  motor_dynamics : simulink_extras/Additional Linear/Transfer Fcn (with initial outputs)  N=[1]  D="[tau_em  1]"  Y0=-tau_m  U0=-tau_m
  TrqOut : Outport
  wires:
  TrqIn/1 -> motor_dynamics/1
  motor_dynamics/1 -> TrqOut/1

== system DemonstratorSimscape/EM System/Motor Winch Left/Motor/Motor with efficiency ==
  MotTrqRef : Inport
  MotSpd : Inport  Port=2
  Divide : Product  Inputs=**
  Gain : Gain  Gain=-1
  Power : Math  Operator=pow  SaturateOnIntegerOverflow=on
  Product1 : Product
  Sign : Signum
  VSD efficiency : Constant  Value=VSD.eff
  motor efficiency : Constant  Value=M.eff
  MotTrq : Outport
  wires:
  Power/1 -> Divide/2
  motor efficiency/1 -> Product1/1
  VSD efficiency/1 -> Product1/2
  Sign/1 -> Power/2
  Divide/1 -> MotTrq/1
  Product1/1 -> Power/1
  MotTrqRef/1 -> Divide/1
  MotSpd/1 -> Gain/1
  Gain/1 -> Sign/1

== system DemonstratorSimscape/EM System/Motor Winch Right/Gearbox/Gearbox efficiency ==
  MotTrqRef : Inport
  MotSpd : Inport  Port=2
  Divide : Product  Inputs=**
  Gain : Gain
  Power : Math  Operator=pow  SaturateOnIntegerOverflow=on
  Sign1 : Signum
  gearbox efficiency : Constant  Value=GB.eff
  WinchTrq : Outport
  wires:
  Power/1 -> Divide/2
  Divide/1 -> WinchTrq/1
  MotTrqRef/1 -> Divide/1
  gearbox efficiency/1 -> Power/1
  Gain/1 -> Sign1/1
  Sign1/1 -> Power/2
  MotSpd/1 -> Gain/1

== system DemonstratorSimscape/EM System/Motor Winch Right/Gearbox/Sheaves efficiency ==
  WinchTrq : Inport
  MotSpd : Inport  Port=2
  Divide : Product  Inputs=**
  Gain : Gain
  Power : Math  Operator=pow  SaturateOnIntegerOverflow=on
  Sign : Signum
  combined sheaves efficiency : Constant  Value=P.eff
  swSheavesEff : ManualSwitch  CurrentSetting=0
  WinchTrq' : Outport
  wires:
  Power/1 -> Divide/2
  Sign/1 -> Power/2
  WinchTrq/1 -> swSheavesEff/1, Divide/1
  combined sheaves efficiency/1 -> Power/1
  Gain/1 -> Sign/1
  MotSpd/1 -> Gain/1
  Divide/1 -> swSheavesEff/2
  swSheavesEff/1 -> WinchTrq'/1

== system DemonstratorSimscape/EM System/Motor Winch Right/Motor/Ideal motor ==
  MotTrqRef : Inport
  MotSpd : Inport  Port=2
  MotTrq : Outport
  wires:
  MotTrqRef/1 -> MotTrq/1

== system DemonstratorSimscape/EM System/Motor Winch Right/Motor/Motor dynamics ==
  TrqIn : Inport
  motor_dynamics : simulink_extras/Additional Linear/Transfer Fcn (with initial outputs)  N=[1]  D="[tau_em  1]"  Y0=-tau_m  U0=-tau_m
  TrqOut : Outport
  wires:
  TrqIn/1 -> motor_dynamics/1
  motor_dynamics/1 -> TrqOut/1

== system DemonstratorSimscape/EM System/Motor Winch Right/Motor/Motor with efficiency ==
  MotTrqRef : Inport
  MotSpd : Inport  Port=2
  Divide : Product  Inputs=**
  Gain : Gain
  Power : Math  Operator=pow  SaturateOnIntegerOverflow=on
  Product1 : Product
  Sign : Signum
  VSD efficiency : Constant  Value=VSD.eff
  motor efficiency : Constant  Value=M.eff
  MotTrq : Outport
  wires:
  Power/1 -> Divide/2
  motor efficiency/1 -> Product1/1
  VSD efficiency/1 -> Product1/2
  Sign/1 -> Power/2
  Divide/1 -> MotTrq/1
  Product1/1 -> Power/1
  MotTrqRef/1 -> Divide/1
  MotSpd/1 -> Gain/1
  Gain/1 -> Sign/1

== system DemonstratorSimscape/Transmission System/Anchor and Load/FlexDisp_Left/L_12 ==
  L(t)[m] : Inport
  a[m/s^2] : Inport  Port=2
  Constant : Constant  Value=C.EA
  Constant1 : Constant  Value=C.dr
  Constant2 : Constant  Value=Part.m
  Constant3 : Constant  Value=g
  Constant4 : Constant  Value=C.drK
  Gain : Gain  Gain=1/Part.m
  Integrator : Integrator
  Integrator1 : Integrator
  Product : Product  Inputs=*/
  Product{1..3,5} (4 alike) : Product
  Product4 : Product  Inputs=*/
  Product6 : Product  Inputs=/*
  SW_b : ManualSwitch  CurrentSetting=0
  Sqrt : Sqrt  SaturateOnIntegerOverflow=on
  Sum1 : Sum  Inputs=+++
  Sum2 : Sum  Inputs=-+
  F[N] : Outport  VectorParamsAs1DForOutWhenUnconnected=off
  ext [m] : Outport  Port=2  VectorParamsAs1DForOutWhenUnconnected=off
  ext speed [m/s] : Outport  Port=3  VectorParamsAs1DForOutWhenUnconnected=off
  wires:
  L(t)[m]/1 -> Product/2
  Constant/1 -> Product/1
  Product2/1 -> Sum1/1
  Product3/1 -> Sum1/3
  Sum2/1 -> Product4/1, F[N]/1
  Product/1 -> Product2/2, Gain/1  "k"
  Constant2/1 -> Product4/2, Product5/2, Product3/2
  Integrator/1 -> ext speed [m/s]/1, Product1/2, Integrator1/1
  Integrator1/1 -> Product2/1, ext [m]/1
  Product4/1 -> Integrator/1
  Product1/1 -> Sum1/2
  a[m/s^2]/1 -> Product3/1
  Sum1/1 -> Sum2/1
  Product5/1 -> Sum2/2
  Constant3/1 -> Product5/1
  Gain/1 -> Sqrt/1
  Sqrt/1 -> Product6/1
  Constant4/1 -> Product6/2
  Constant1/1 -> SW_b/2
  Product6/1 -> SW_b/1
  SW_b/1 -> Product1/1
